simulink model "oppg3"  (R2021b)
settings: Solver=VariableStepAuto  StartTime=0.0  StopTime=2400  RelTol=1e-3
settings Model: Creator=rezoa  LastModifiedBy=rezoan
settings SolverCC: AlgebraicLoopSolver=TrustRegion
settings DebuggingCC: SFMachineParentedDataDiag=warning

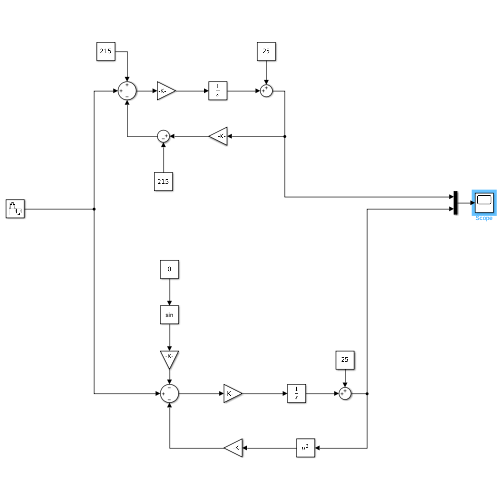
[thumbnail: Simulink's stored preview of the top-level diagram]
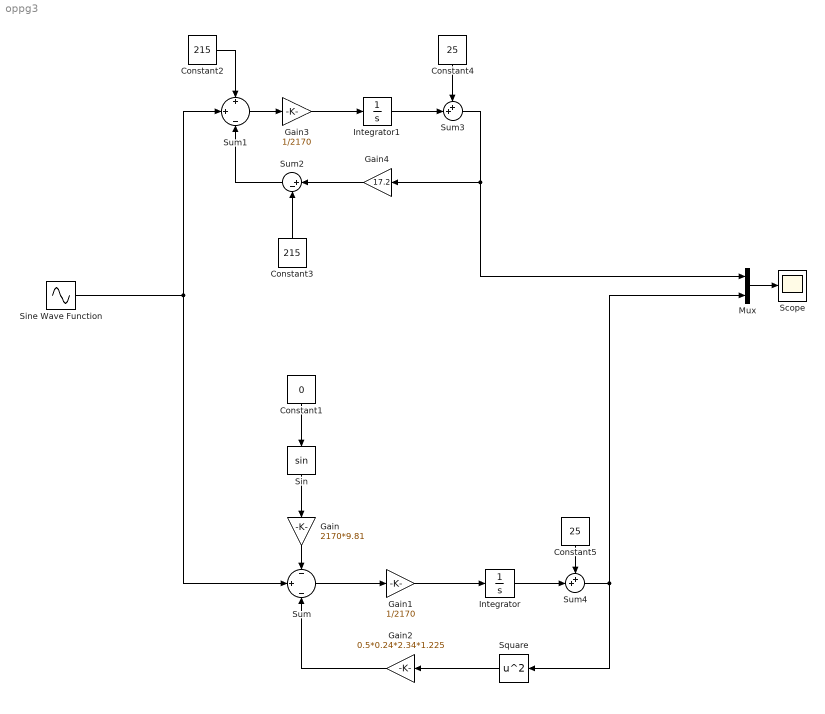
== system oppg3 ==
  Constant1 : Constant  Value=0
  Constant2 : Constant  Value=215
  Constant3 : Constant  Value=215
  Constant4 : Constant  Value=25
  Constant5 : Constant  Value=25
  Gain : Gain  Gain=2170*9.81
  Gain1 : Gain  Gain=1/2170
  Gain2 : Gain  Gain=0.5*0.24*2.34*1.225
  Gain3 : Gain  Gain=1/2170
  Gain4 : Gain  Gain=17.2
  Integrator : Integrator
  Integrator1 : Integrator
  Mux : Mux  Inputs=2
  Scope : Scope
  Sin : Trigonometry
  Sine Wave Function : Sin  Amplitude=5000  Frequency=(2*pi)/30  SampleTime=0.001
  Square : Math  Operator=square  SaturateOnIntegerOverflow=on
  Sum : Sum  Inputs=-|+|-
  Sum1 : Sum  Inputs=+|+|-
  Sum2 : Sum  Inputs=|+-
  Sum3 : Sum  Inputs=++|
  Sum4 : Sum  Inputs=++|
  wires:
  Constant1/1 -> Sin/1
  Sin/1 -> Gain/1
  Gain/1 -> Sum/1
  Sine Wave Function/1 -> Sum1/2, Sum/2
  Sum/1 -> Gain1/1
  Gain1/1 -> Integrator/1
  Square/1 -> Gain2/1
  Gain2/1 -> Sum/3
  Constant2/1 -> Sum1/1
  Sum1/1 -> Gain3/1
  Gain3/1 -> Integrator1/1
  Gain4/1 -> Sum2/1
  Constant3/1 -> Sum2/2
  Integrator1/1 -> Sum3/2
  Sum3/1 -> Mux/1, Gain4/1
  Constant4/1 -> Sum3/1
  Integrator/1 -> Sum4/2
  Sum4/1 -> Mux/2, Square/1
  Constant5/1 -> Sum4/1
  Mux/1 -> Scope/1
  Sum2/1 -> Sum1/3
